simulink model "PassVeh7DOF"  (R2024b)
settings: Solver=ode14x  StartTime=0.0  StopTime=30  FixedStep=0.001  RelTol=1e-1
model workspace (MAT data in the model file):
  A_mu = 10
  B_reff = 8.386
  CONVERTER_DATA = [0 0.1 0.2 0.3 0.4 0.5 0.6 0.7 0.8 0.81 0.82 0.83 ... (63 elements, 21x3)]
  Cps = 2
  Cz = 7766.25
  DOWN_TABLE = [0 0 0 0 0 0 5 5 7.5 7.5 15 15 ... (30 elements, 6x5)]
  DOWN_TH_BP = [0 5 40 50 90 100]
  D_reff = 0.25826
  EMAP = [-40 215 245 264 264 267 267 267 267 267 -44 117 ... (110 elements, 10x11)]
  F0z = [6086.4 4324.8]
  F_reff = 0.07394
  F_zmax = 10000
  F_zmin = 100
  F_zo = 4000
  Kz = 48000
  MF : object (value not decoded)
  NCyl = 6
  NE_VEC = [800 1200 1600 2000 2400 2800 3200 3600 4000 4400 4800]
  Pstd = 101325
  R_eff = 0.298
  Rair = 287
  SUS : object (value not decoded)
  TH_VEC = [0; 20; 30; 40; 50; 60; 70; 80; 90; 100]
  TWAITdn = 1.25
  TWAITup = 0.1
  Tin = [1 2 3 4 5 6 7 8 9 10 2 2 ... (20 elements, 10x2)]
  Tstd = 293.15
  UP_TABLE = [7.5 7.5 15 25 40 40 25 25 35 45 70 80 ... (30 elements, 6x5)]
  UP_TH_BP = [0 25 35 50 90 100]
  VEH : object (value not decoded)
  V_o = 16.7
  V_xlow = 1
  Vd = 0.00346
  WH : object (value not decoded)
  a = 1.515
  alpha_max = 1.5
  alpha_min = -1.5
  b = 1.504
  c_zo = 209651
  epsilon = 0.1
  f_air = [0 0 0 0 0 0 0 0 0 0 0 0 ... (256 elements, 16x16)]
  f_co = [0 0 0 0 0 0 0 0 0 0 0 0 ... (256 elements, 16x16)]
  f_co2 = [0 0 0 0 0 0 0 0 0 0 0 0 ... (256 elements, 16x16)]
  f_eff = [352.135682859 352.135682859 320.724378192 303.655312657 295.930136708 291.240087194 291.240271258 291.240312459 291.240275452 291.240198499 291.240100781 291.240018769 ... (256 elements, 16x16)]
  f_fuel = [0 0 0 0 0 0 0 0 0 0 0 0 ... (256 elements, 16x16)]
  f_hc = [0 0 0 0 0 0 0 0 0 0 0 0 ... (256 elements, 16x16)]
  f_nox = [0 0 0 0 0 0 0 0 0 0 0 0 ... (256 elements, 16x16)]
  f_pm = [0 0 0 0 0 0 0 0 0 0 0 0 ... (256 elements, 16x16)]
  f_susp_axl_bp = [1 2]
  f_susp_dz_bp = [-4 -0.14 -0.13 -0.12 -0.11 -0.1 -0.09 -0.08 -0.07 -0.06 -0.05 -0.04 ... (31 elements, 1x31)]
  f_susp_dzdot_bp = [-4 -0.14 -0.13 -0.12 -0.11 -0.1 -0.09 -0.08 -0.07 -0.06 -0.05 -0.04 ... (31 elements, 1x31)]
  f_susp_fmz = [-213379.591456 -28099.591456 -27619.591456 -27139.591456 -26659.591456 -26179.591456 -25699.591456 -25219.591456 -24739.591456 -24259.591456 -23779.591456 -23299.591456 ... (468968 elements, 31x31x61x2x4)]
  f_susp_geom = [-0.832564012244 0.043269987756 0.045538987756 0.047807987756 0.050076987756 0.052345987756 0.054614987756 0.056883987756 0.059152987756 0.061421987756 0.063690987756 0.065959987756 ... (11346 elements, 31x61x2x3)]
  f_susp_strgdelta_bp = [-0.523598775598 -0.506145483078 -0.488692190558 -0.471238898038 -0.453785605519 -0.436332312999 -0.418879020479 -0.401425727959 -0.383972435439 -0.366519142919 -0.349065850399 -0.331612557879 ... (61 elements, 1x61)]
  f_tbrake = [0 76.8593923996 105.140482948 131.533638111 157.926793274 176.658631717 176.65727296 176.656856686 176.656879077 176.657093756 176.657404516 176.65772406 ... (256 elements, 16x16)]
  f_tbrake_n_bpt = [0 649.519052838 912.419621844 1175.32019085 1438.22075986 1701.12132886 1964.02189787 2226.92246687 2489.82303588 2752.72360489 3015.62417389 3278.5247429 ... (16 elements, 1x16)]
  f_tbrake_t_bpt = [0 34.6410161514 61.0341713143 87.4273264773 113.82048164 140.213636803 166.606791966 192.999947129 219.393102292 245.786257455 272.179412618 298.572567781 ... (16 elements, 1x16)]
  f_texh = [766.752464599 766.752464599 786.17542386 801.679939032 884.591982581 910.574397722 910.571871054 910.570774534 910.570601632 910.570821151 910.571247242 910.571639815 ... (256 elements, 16x16)]
  f_twc_eff_co = [0.17 0.25 0.45 0.99 0.99 0.99 0.99]
  f_twc_eff_hc = [0.21 0.375 0.75 0.98 0.98 0.98 0.98]
  f_twc_eff_lam = [0.909090909 0.944055944 0.979020979 1 1.013986014 1.048951049 1.083916084]
  f_twc_eff_nox = [0.98 0.98 0.98 0.97 0.05 0.02 0]
  h = 0.134
  k_z = 50
  kappa_max = 1.5
  kappa_min = -1.5
  lam_Cx = 1
  lam_Cy = 1
  lam_Cz = 1
  lam_Ex = 1
  lam_Ey = 1
  lam_F_zo = 1
  lam_Hx = 1
  lam_Hy = 1
  lam_Kxkappa = 1
  lam_Kyalpha = 1
  lam_Kygamma = 1
  lam_Kzgamma = 1
  lam_Mr = 1
  lam_Mx = 1
  lam_My = 1
  lam_S = 1
  lam_VMx = 1
  lam_Vx = 1
  lam_Vy = 1
  lam_Vykappa = 1
  lam_muV = 0
  lam_mux = 1
  lam_muy = 1
  lam_t = 1
  lam_xalpha = 1
  lam_ykappa = 1
  numWheel = 4
  p_Cx1 = 1.579
  p_Cy1 = 1.3332
  p_Dx1 = 1.0422
  p_Dx2 = -0.08285
  p_Dx3 = 0
  p_Dy1 = 0.8784
  p_Dy2 = -0.06445
  p_Dy3 = 0
  p_Ex1 = 0.11185
  p_Ex2 = 0.3127
  p_Ex3 = 0
  p_Ex4 = 0.001603
  p_Ey1 = -0.8227
  p_Ey2 = -0.6062
  p_Ey3 = 0.09825
  p_Ey4 = -6.546
  p_Ey5 = 0
  p_Fz1 = 0.7098
  p_Hx1 = 0.00021585
  p_Hx2 = 0.0011538
  p_Hy1 = -0.0018043
  p_Hy2 = 0.003518
  p_Kx1 = 21.69
  p_Kx2 = 13.774
  p_Kx3 = -0.4119
  p_Ky1 = -15.314
  p_Ky2 = 1.7044
  p_Ky3 = 0.36986
  p_Ky4 = 1.9896
  p_Ky5 = 0
  p_Ky6 = -0.9004
  p_Ky7 = -0.2328
  p_Vx1 = 1.5973e-05
  p_Vx2 = 0.0001043
  p_Vy1 = -0.006642
  p_Vy2 = 0.03597
  p_Vy3 = -0.1621
  p_Vy4 = -0.4908
  p_pmx1 = 0
  p_px1 = -0.3489
  p_px2 = 0.382
  p_px3 = -0.09634
  p_px4 = 0.06447
  p_py1 = -0.6249
  p_py2 = -0.06535
  p_py3 = -0.1668
  p_py4 = 0.2834
  p_py5 = 0
  path : object (value not decoded)
  pio = 220000
  q_Fcx = 0
  q_Fz2 = 15.4
  q_Fzy = 0
  q_reo = 0.9974
  q_sx1 = -0.007764
  q_sx10 = 0.2824
  q_sx11 = 5.349
  q_sx12 = 0
  q_sx13 = 0
  q_sx14 = 0
  q_sx2 = 1.1915
  q_sx3 = 0.013948
  q_sx4 = 4.912
  q_sx5 = 1.02
  q_sx6 = 22.83
  q_sx7 = 0.7104
  q_sx8 = -0.023393
  q_sx9 = 0.6581
  q_sy1 = 0.00702
  q_sy2 = 0
  q_sy3 = 0.001515
  q_sy4 = 8.514e-05
  q_sy5 = 0
  q_sy6 = 0
  q_sy7 = 0.9008
  q_sy8 = -0.4089
  q_v1 = 0.0007742
  q_v2 = 0.04667
  r_Bx1 = 12.531
  r_Bx2 = 9.532
  r_Bx3 = 0
  r_By1 = 10.615
  r_By2 = 7.705
  r_By3 = 3.433e-06
  r_By4 = 0
  r_Cx1 = 1.019
  r_Cy1 = 1.0585
  r_Ex1 = -0.4487
  r_Ex2 = -0.4726
  r_Ey1 = 0.3132
  r_Ey2 = 7.63e-06
  r_Hx1 = 0.0002374
  r_Hy1 = 0.011646
  r_Hy2 = 7.63e-06
  r_Vy1 = 0.05654
  r_Vy2 = 7.63e-06
  r_Vy3 = 0
  r_Vy4 = 99.9
  r_Vy5 = 2
  r_Vy6 = 15.814
  r_o = 0.3135
  reqTmaxT = [nan 0.285774810084 0.647179872268 nan nan nan nan nan nan nan nan nan ... (168 elements, 21x8)]
  vehSpd = [0 2.77777777778 5.55555555556 8.33333333333 11.1111111111 13.8888888889 16.6666666667 19.4444444444 22.2222222222 25 27.7777777778 30.5555555556 ... (21 elements, 1x21)]
  vehWidth = 2
  w = 1
symbols that are objects in the model workspace (value not decoded): VEH
undefined symbols (not defined in the file or in its folder): Fzz, Fzzdot, InertFrm, pFz, psi, vdyntiremask, x_o, zdotFz, zFz
libraries: simulink x4, sharedTrackingLibrary x1, mcbcontrolslib x1
(part 8 of 24)

== system PassVeh7DOF/Longitudinal Wheels 4DOF/Tires/Fiala/Fiala Tire/Vertical DOF ==
  "GroundInput " : Inport
  "Fext " : Inport  Port=2
  rho : Inport  Port=3
  "GndFz " : Inport  Port=4
  Prs : Inport  Port=5
  External : Subsystem  VariantControl=vertType==3
  Mapped Vertical DOF : Subsystem  VariantControl=vertType==2
  None : Subsystem  VariantControl=vertType==1
  Vertical Wheel and Unsprung Mass Response : Subsystem  VariantControl=vertType==4  mask{m=MASS, bz=VERTICAL_DAMPING, zo=zo, zdoto=zdoto, g=GRAVITY, ReMax=UNLOADED_RADIUS}
      mask prompts: m "Unsprung mass [kg]"; bz "Vertical damping [N*m/s]"; zo "Initial deflection [m]"; zdoto "Initial velocity [m/s]"; g "Gravitational acceleration [m/s^2]"; ReMax "Maximum unloaded radius [m]:"
  RadialDeflct : Outport  VectorParamsAs1DForOutWhenUnconnected=off
  " z" : Outport  Port=2  VectorParamsAs1DForOutWhenUnconnected=off
  " zdot" : Outport  Port=3  VectorParamsAs1DForOutWhenUnconnected=off
  GndFz : Outport  Port=4  VectorParamsAs1DForOutWhenUnconnected=off

== system PassVeh7DOF/Longitudinal Wheels 4DOF/Tires/Fiala/Fiala Tire/Wheel Module ==
  BrkPrs : Inport
  AxlTrq : Inport  Port=2
  TireFdbk : Inport  Port=3
  RadialDeflct : Inport  Port=4
  Add1 : Sum  Inputs=--+
  Add2 : Sum  Inputs=-+
  Brakes : Subsystem  Variant=on  VariantControlMode=label  LabelModeActiveChoice=Disk  mask{aMode=aMode}
  Bus Selector1 : BusSelector  OutputSignals=My,Fx
  Clutch : Subsystem  Variant=on  VariantControlMode=label  VariantControl=Choice  LabelModeActiveChoice=0
  Constant9 : Constant  Value=UNLOADED_RADIUS
  Friction Model : Subsystem
  Product3 : Product  Inputs=**
  Reshape : Reshape
  Saturation : Saturate  UpperLimit=inf  LowerLimit=0  ZeroCross=off
  Terminator1 : Terminator
  Terminator3 : Terminator
  MyBrk : Outport  VectorParamsAs1DForOutWhenUnconnected=off
  Omega : Outport  Port=2  VectorParamsAs1DForOutWhenUnconnected=off
  wires:
  Reshape/1 -> Clutch/1(Tout)
  Product3/1 -> Add1/3
  AxlTrq/1 -> Add1/1
  RadialDeflct/1 -> Add2/1
  Friction Model/2(Tfmaxk) -> Clutch/3(Tfmaxk)
  Friction Model/1(Tfmaxs) -> Clutch/2(Tfmaxs)
  Add1/1 -> Reshape/1
  Clutch/3(Myb) -> Terminator1/1
  Clutch/2(Omegadot) -> Terminator3/1
  Clutch/1(Omega) -> Brakes/2(Omega), Omega/1
  Saturation/1 -> Product3/2
  Brakes/1(MyBrk) -> Friction Model/1(Brake torque), MyBrk/1
  Add2/1 -> Saturation/1
  Constant9/1 -> Add2/2
  BrkPrs/1 -> Brakes/1(BrkPrs)
  Bus Selector1/2 -> Product3/1  "<Fx>"
  Bus Selector1/1 -> Add1/2  "<My>"
  TireFdbk/1 -> Bus Selector1/1

== system PassVeh7DOF/Longitudinal Wheels 4DOF/Tires/MF/Combined Slip Wheel 2DOF/Bus Routing ==
  BrkPrs : Inport
  BrkTrq : Inport  Port=2
  omega : Inport  Port=3
  FLong : Inport  Port=4
  Flat : Inport  Port=5
  FzTire : Inport  Port=6
  MOver : Inport  Port=7
  MRoll : Inport  Port=8
  MAlign : Inport  Port=9
  Re : Inport  Port=10
  Kappa : Inport  Port=11
  Alpha : Inport  Port=12
  a : Inport  Port=13
  b : Inport  Port=14
  RL : Inport  Port=15
  RadialDeflct : Inport  Port=16
  WhlTrq : Inport  Port=17
  z : Inport  Port=18
  zdot : Inport  Port=19
  AxlTrq : Inport  Port=20
  Vx : Inport  Port=21
  Vy : Inport  Port=22
  Gamma : Inport  Port=23
  psidot : Inport  Port=24
  Prs : Inport  Port=25
  Gnd : Inport  Port=26
  FNormal : Inport  Port=27
  Bus Creator : BusCreator  Inputs=27
  Signal Copy : SignalConversion  OverrideOpt=off
  Signal Specification{,3,6..7,22..23} (6 alike) : SignalSpecification  Unit=m
  Signal Specification1 : SignalSpecification  Unit=1
  Signal Specification{5,8,15..17} (5 alike) : SignalSpecification  Unit=N*m
  Signal Specification18 : SignalSpecification  Unit=N
  Signal Specification19 : SignalSpecification  Unit=N
  Signal Specification2 : SignalSpecification  Unit=rad
  Signal Specification20 : SignalSpecification  Unit=N
  Signal Specification21 : SignalSpecification  Unit=rad/s
  Signal Specification4 : SignalSpecification  Unit=m/s
  Info : Outport  VectorParamsAs1DForOutWhenUnconnected=off
  Omega : Outport  Port=2  Unit=rad/s  VectorParamsAs1DForOutWhenUnconnected=off
  Fx : Outport  Port=3  Unit=N  VectorParamsAs1DForOutWhenUnconnected=off
  Fy : Outport  Port=4  Unit=N  VectorParamsAs1DForOutWhenUnconnected=off
  Fz : Outport  Port=5  Unit=N  VectorParamsAs1DForOutWhenUnconnected=off
  Mx : Outport  Port=6  Unit=N*m  VectorParamsAs1DForOutWhenUnconnected=off
  My : Outport  Port=7  Unit=N*m  VectorParamsAs1DForOutWhenUnconnected=off
  Mz : Outport  Port=8  Unit=N*m  VectorParamsAs1DForOutWhenUnconnected=off
  wires:
  Signal Specification5/1 -> Bus Creator/21  "BrkTrq"
  psidot/1 -> Bus Creator/20  "psidot"
  Gamma/1 -> Bus Creator/19  "Gamma"
  Signal Specification8/1 -> Bus Creator/18  "WhlTrq"
  Signal Specification7/1 -> Bus Creator/17  "RadialDeflct"
  Signal Specification6/1 -> Bus Creator/16  "RL"
  RL/1 -> Signal Specification6/1
  RadialDeflct/1 -> Signal Specification7/1
  WhlTrq/1 -> Signal Specification8/1
  MRoll/1 -> Signal Specification16/1
  FzTire/1 -> Signal Copy/1
  Signal Copy/1 -> Signal Specification18/1
  Prs/1 -> Bus Creator/27  "Prs"
  Gnd/1 -> Bus Creator/25  "Gnd"
  Signal Specification18/1 -> Bus Creator/26  "GndFz"
  BrkPrs/1 -> Bus Creator/22  "BrkPrs"
  Vy/1 -> Bus Creator/10  "Vy"
  Vx/1 -> Bus Creator/9  "Vx"
  AxlTrq/1 -> Bus Creator/1  "AxlTrq"
  BrkTrq/1 -> Signal Specification5/1
  Kappa/1 -> Signal Specification1/1
  z/1 -> Signal Specification3/1
  zdot/1 -> Signal Specification4/1
  Re/1 -> Signal Specification/1
  b/1 -> Signal Specification22/1
  Flat/1 -> Signal Specification19/1
  MAlign/1 -> Signal Specification15/1
  Signal Specification22/1 -> Bus Creator/15  "b"
  Signal Specification23/1 -> Bus Creator/14  "a"
  Signal Specification20/1 -> Fx/1, Bus Creator/3  "Fx"
  Signal Specification2/1 -> Bus Creator/13  "Alpha"
  omega/1 -> Signal Specification21/1
  Signal Specification16/1 -> Bus Creator/7, My/1  "My"
  Signal Specification19/1 -> Bus Creator/4, Fy/1  "Fy"
  FLong/1 -> Signal Specification20/1
  Signal Specification1/1 -> Bus Creator/12  "Kappa"
  MOver/1 -> Signal Specification17/1
  Signal Specification17/1 -> Bus Creator/6, Mx/1  "Mx"
  Bus Creator/1 -> Info/1
  Signal Specification/1 -> Bus Creator/11  "Re"
  Signal Specification15/1 -> Bus Creator/8, Mz/1  "Mz"
  FNormal/1 -> Bus Creator/5, Fz/1  "Fz"
  Signal Specification21/1 -> Omega/1, Bus Creator/2  "Omega"
  Signal Specification4/1 -> Bus Creator/24  "zdot"
  Alpha/1 -> Signal Specification2/1
  a/1 -> Signal Specification23/1
  Signal Specification3/1 -> Bus Creator/23  "z"

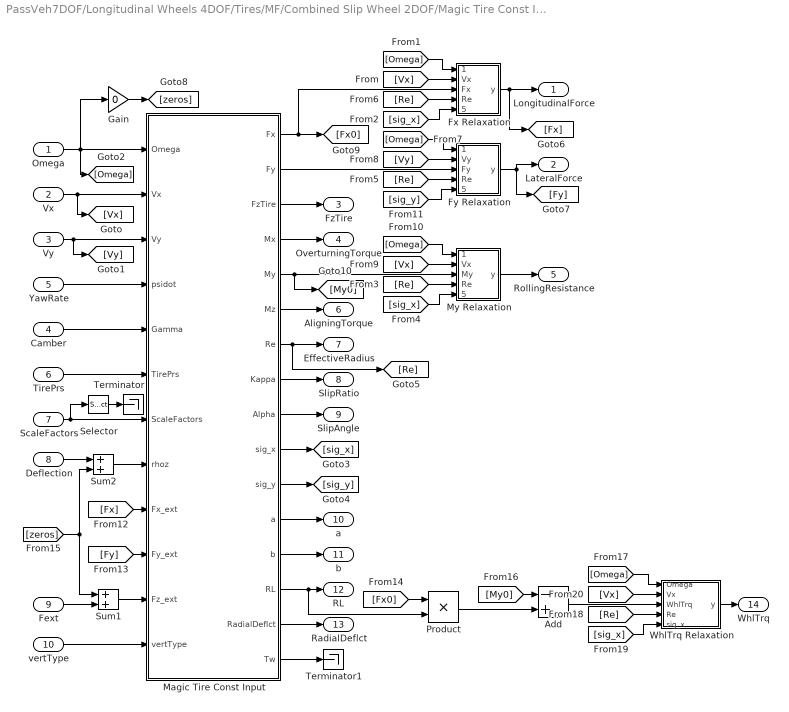
== system PassVeh7DOF/Longitudinal Wheels 4DOF/Tires/MF/Combined Slip Wheel 2DOF/Magic Tire Const Input ==
  Omega : Inport
  Vx : Inport  Port=2
  Vy : Inport  Port=3
  Camber : Inport  Port=4
  YawRate : Inport  Port=5
  TirePrs : Inport  Port=6
  ScaleFactors : Inport  Port=7
  Deflection : Inport  Port=8
  Fext : Inport  Port=9
  vertType : Inport  Port=10
  Add : Sum  Inputs=-+
  Fx Relaxation : Subsystem
  Fy Relaxation : Subsystem
  Gain : Gain  Gain=0
  Magic Tire Const Input : MATLAB Function
  My Relaxation : Subsystem
  Product : Product
  Selector : Selector  NumberOfDimensions=2  InputPortWidth=3  IndexOptions=Index vector (dialog),Select all  Indices=[1:27],1  OutputSizes=1,1
  Sum1 : Sum
  Sum2 : Sum
  Terminator : Terminator
  Terminator1 : Terminator
  WhlTrq Relaxation : Subsystem
  LongitudinalForce : Outport  VectorParamsAs1DForOutWhenUnconnected=off
  LateralForce : Outport  Port=2  VectorParamsAs1DForOutWhenUnconnected=off
  FzTire : Outport  Port=3  VectorParamsAs1DForOutWhenUnconnected=off
  OverturningTorque : Outport  Port=4  VectorParamsAs1DForOutWhenUnconnected=off
  RollingResistance : Outport  Port=5  VectorParamsAs1DForOutWhenUnconnected=off
  AligningTorque : Outport  Port=6  VectorParamsAs1DForOutWhenUnconnected=off
  EffectiveRadius : Outport  Port=7  VectorParamsAs1DForOutWhenUnconnected=off
  SlipRatio : Outport  Port=8  VectorParamsAs1DForOutWhenUnconnected=off
  SlipAngle : Outport  Port=9  VectorParamsAs1DForOutWhenUnconnected=off
  a : Outport  Port=10  VectorParamsAs1DForOutWhenUnconnected=off
  b : Outport  Port=11  VectorParamsAs1DForOutWhenUnconnected=off
  RL : Outport  Port=12
  RadialDeflct : Outport  Port=13
  WhlTrq : Outport  Port=14
  wires:
  Add/1 -> WhlTrq Relaxation/3(WhlTrq)
  WhlTrq Relaxation/1(y) -> WhlTrq/1
  [Re] -> WhlTrq Relaxation/4(Re)
  [Vx] -> WhlTrq Relaxation/2(Vx)
  [sig_x] -> WhlTrq Relaxation/5(sig_x)
  [Omega] -> WhlTrq Relaxation/1(Omega)
  [My0] -> Add/1
  Deflection/1 -> Sum2/1
  Sum2/1 -> Magic Tire Const Input/8(rhoz)
  [zeros] -> Sum2/2, Sum1/1
  Sum1/1 -> Magic Tire Const Input/11(Fz_ext)
  Fext/1 -> Sum1/2
  Gain/1 -> [zeros]
  Product/1 -> Add/2
  [Fx0] -> Product/1
  Magic Tire Const Input/16(Tw) -> Terminator1/1
  Magic Tire Const Input/15(RadialDeflct) -> RadialDeflct/1
  Magic Tire Const Input/14(RL) -> RL/1, Product/2
  Selector/1 -> Terminator/1
  vertType/1 -> Magic Tire Const Input/12(vertType)
  [Fy] -> Magic Tire Const Input/10(Fy_ext)
  [Fx] -> Magic Tire Const Input/9(Fx_ext)
  Magic Tire Const Input/1(Fx) -> [Fx0], Fx Relaxation/3(Fx)
  [sig_y] -> Fy Relaxation/5(sig_y)
  [Omega] -> My Relaxation/1(Omega)
  [Vx] -> My Relaxation/2(Vx)
  [Vy] -> Fy Relaxation/2(Vy)
  [Omega] -> Fy Relaxation/1(Omega)
  [Re] -> Fx Relaxation/4(Re)
  [Re] -> Fy Relaxation/4(Re)
  [sig_x] -> My Relaxation/5(sig_x)
  [Re] -> My Relaxation/4(Re)
  [sig_x] -> Fx Relaxation/5(sig_x)
  Magic Tire Const Input/11(sig_y) -> [sig_y]
  Magic Tire Const Input/10(sig_x) -> [sig_x]
  [Omega] -> Fx Relaxation/1(Omega)
  [Vx] -> Fx Relaxation/2(Vx)
  Fy Relaxation/1(y) -> [Fy], LateralForce/1
  Magic Tire Const Input/12(a) -> a/1
  Magic Tire Const Input/13(b) -> b/1
  Magic Tire Const Input/5(My) -> My Relaxation/3(My), [My0]
  Vy/1 -> Magic Tire Const Input/3(Vy), [Vy]
  Vx/1 -> [Vx], Magic Tire Const Input/2(Vx)
  My Relaxation/1(y) -> RollingResistance/1
  Fx Relaxation/1(y) -> [Fx], LongitudinalForce/1
  Magic Tire Const Input/7(Re) -> [Re], EffectiveRadius/1
  Magic Tire Const Input/2(Fy) -> Fy Relaxation/3(Fy)
  Magic Tire Const Input/9(Alpha) -> SlipAngle/1
  Magic Tire Const Input/8(Kappa) -> SlipRatio/1
  Magic Tire Const Input/6(Mz) -> AligningTorque/1
  Magic Tire Const Input/4(Mx) -> OverturningTorque/1
  ScaleFactors/1 -> Selector/1, Magic Tire Const Input/7(ScaleFactors)
  TirePrs/1 -> Magic Tire Const Input/6(TirePrs)
  Camber/1 -> Magic Tire Const Input/5(Gamma)
  YawRate/1 -> Magic Tire Const Input/4(psidot)
  Omega/1 -> [Omega], Magic Tire Const Input/1(Omega), Gain/1
  Magic Tire Const Input/3(FzTire) -> FzTire/1

== system PassVeh7DOF/Longitudinal Wheels 4DOF/Tires/MF/Combined Slip Wheel 2DOF/Vertical DOF ==
  "GroundInput " : Inport
  "Fext " : Inport  Port=2
  rho : Inport  Port=3
  Prs : Inport  Port=4
  Omega : Inport  Port=5
  Gamma : Inport  Port=6
  Fx_ext : Inport  Port=7
  Fy_ext : Inport  Port=8
  "GndFz " : Inport  Port=9
  ScaleFctrs : Inport  Port=10
  External : Subsystem  VariantControl=vertType==3
  Mapped Vertical DOF : Subsystem  VariantControl=vertType==4
  None : Subsystem  VariantControl=vertType==1
  Vertical Wheel and Unsprung Mass Response : Subsystem  VariantControl=vertType==2  mask{m=MASS, bz=VERTICAL_DAMPING, zo=zo, zdoto=zdoto, g=GRAVITY, ReMax=UNLOADED_RADIUS}
      mask prompts: m "Unsprung mass [kg]"; bz "Vertical damping [N*m/s]"; zo "Initial deflection [m]"; zdoto "Initial velocity [m/s]"; g "Gravitational acceleration [m/s^2]"; ReMax "Maximum unloaded radius [m]:"
  " RadialDeflct" : Outport  VectorParamsAs1DForOutWhenUnconnected=off
  GndFz : Outport  Port=2  VectorParamsAs1DForOutWhenUnconnected=off
  " z" : Outport  Port=3  VectorParamsAs1DForOutWhenUnconnected=off
  " zdot" : Outport  Port=4  VectorParamsAs1DForOutWhenUnconnected=off

== system PassVeh7DOF/Longitudinal Wheels 4DOF/Tires/MF/Combined Slip Wheel 2DOF/Wheel Module ==
  BrkPrs : Inport
  AxlTrq : Inport  Port=2
  TireFdbk : Inport  Port=3
  RadialDeflct : Inport  Port=4
  Add1 : Sum  Inputs=--+
  Add2 : Sum  Inputs=-+
  Brakes : Subsystem  Variant=on  VariantControlMode=label  LabelModeActiveChoice=Disk  mask{aMode=aMode}
  Bus Selector1 : BusSelector  OutputSignals=My,Fx
  Clutch : Subsystem  Variant=on  VariantControlMode=label  VariantControl=Choice  LabelModeActiveChoice=0
  Constant9 : Constant  Value=UNLOADED_RADIUS
  Friction Model : Subsystem
  Product3 : Product  Inputs=**
  Reshape : Reshape
  Saturation : Saturate  UpperLimit=inf  LowerLimit=0  ZeroCross=off
  Terminator1 : Terminator
  Terminator3 : Terminator
  MyBrk : Outport  VectorParamsAs1DForOutWhenUnconnected=off
  Omega : Outport  Port=2  VectorParamsAs1DForOutWhenUnconnected=off
  wires:
  Reshape/1 -> Clutch/1(Tout)
  Product3/1 -> Add1/3
  AxlTrq/1 -> Add1/1
  RadialDeflct/1 -> Add2/1
  Friction Model/2(Tfmaxk) -> Clutch/3(Tfmaxk)
  Friction Model/1(Tfmaxs) -> Clutch/2(Tfmaxs)
  Add1/1 -> Reshape/1
  Clutch/3(Myb) -> Terminator1/1
  Clutch/2(Omegadot) -> Terminator3/1
  Clutch/1(Omega) -> Brakes/2(Omega), Omega/1
  Saturation/1 -> Product3/2
  Brakes/1(MyBrk) -> Friction Model/1(Brake torque), MyBrk/1
  Add2/1 -> Saturation/1
  Constant9/1 -> Add2/2
  BrkPrs/1 -> Brakes/1(BrkPrs)
  Bus Selector1/2 -> Product3/1  "<Fx>"
  Bus Selector1/1 -> Add1/2  "<My>"
  TireFdbk/1 -> Bus Selector1/1

== system PassVeh7DOF/Longitudinal Wheels 4DOF/Tires/MF/Combined Slip Wheel 2DOF/a_cmd ==
  note: $\alpha_{\text{cmd}} = \arctan\left( \frac{v_y + ar}{v_x} \right) - \delta$
  Vx : Inport
  Vy : Inport  Port=2
  WhlAng : Inport  Port=3
  YawRate : Inport  Port=4
  Add1 : Sum
  Gain : Gain  Gain=VEH.FrontAxlePositionfromCG
  Subtract : Sum  Inputs=+-
  atan2 : mcbcontrolslib/atan2  ApproximationMethod=None  NumberOfIterations=11  NumberOfDataPoints=16  InterpMethod=Flat  outputUnit=Radians  TableDataTypeStr=Inherit: Inherit via input
      settings: LibrarySourceBlock=mcblib/Controls/Math Transforms/atan2
  alphacmd : Outport
  wires:
  Subtract/1 -> alphacmd/1
  WhlAng/1 -> Subtract/2
  Add1/1 -> atan2/1
  Vy/1 -> Add1/1
  atan2/1 -> Subtract/1
  Gain/1 -> Add1/2
  YawRate/1 -> Gain/1
  Vx/1 -> atan2/2

== system PassVeh7DOF/Longitudinal Wheels 4DOF/Tires/MF/Combined Slip Wheel 2DOF/k_cmd ==
  note: $\kappa_{\text{cmd}} = \frac{R_{\text{eff}} \cdot \omega - v_x}{\max(|v_x|, 0.1)}$$
  Omega : Inport
  Vx : Inport  Port=2
  Abs : Abs  SaturateOnIntegerOverflow=off
  Constant : Constant  Value=0.1
  Divide : Product  Inputs=*/
  Gain : Gain  Gain=R_eff
  Max : MinMax  Function=max  Inputs=2
  Subtract : Sum  Inputs=+-
  k_cmd : Outport
  wires:
  Gain/1 -> Subtract/1
  Omega/1 -> Gain/1
  Max/1 -> Divide/2
  Constant/1 -> Max/2
  Vx/1 -> Subtract/2, Abs/1
  Subtract/1 -> Divide/1
  Abs/1 -> Max/1
  Divide/1 -> k_cmd/1

== system PassVeh7DOF/Longitudinal Wheels 4DOF/Veh2Tire/Wheel to Body Transform/Rotation Angles to Direction Cosine Matrix/Create 3x3 Matrix ==
  M11 : Inport  PortDimensions=1
  M12 : Inport  Port=2  PortDimensions=1
  M13 : Inport  Port=3  PortDimensions=1
  M21 : Inport  Port=4  PortDimensions=1
  M22 : Inport  Port=5  PortDimensions=1
  M23 : Inport  Port=6  PortDimensions=1
  M31 : Inport  Port=7  PortDimensions=1
  M32 : Inport  Port=8  PortDimensions=1
  M33 : Inport  Port=9  PortDimensions=1
  Reshape (9) to [3x3] column-major : Reshape  OutputDimensionality=Customize  OutputDimensions=[3,3]
  Vector Concatenate : Concatenate  NumInputs=9
  Matrix : Outport  PortDimensions=[3 3]  VectorParamsAs1DForOutWhenUnconnected=off
  wires:
  M33/1 -> Vector Concatenate/9
  M23/1 -> Vector Concatenate/8
  M13/1 -> Vector Concatenate/7
  M32/1 -> Vector Concatenate/6
  Reshape (9) to [3x3] column-major/1 -> Matrix/1
  M22/1 -> Vector Concatenate/5
  M12/1 -> Vector Concatenate/4
  M31/1 -> Vector Concatenate/3
  M21/1 -> Vector Concatenate/2
  M11/1 -> Vector Concatenate/1
  Vector Concatenate/1 -> Reshape (9) to [3x3] column-major/1

== system PassVeh7DOF/Longitudinal Wheels 4DOF/Velocity and Vertical Load/Bicycle/Bicycle Fz/Cont LPF ==
  u : Inport
  Constant : Constant  Value=wc
  Divide : Product  Inputs=**
  FixPt Data Type Duplicate1 : DataTypeDuplicate  DisableCoverage=on  NumInputPorts=4
  Integrator1 : Integrator
  Sum : Sum  Inputs=|+-
  y : Outport  VectorParamsAs1DForOutWhenUnconnected=off
  wires:
  Constant/1 -> Divide/2
  [y] -> FixPt Data Type Duplicate1/3
  [wumy] -> FixPt Data Type Duplicate1/4
  [umy] -> FixPt Data Type Duplicate1/2
  [u] -> FixPt Data Type Duplicate1/1
  Integrator1/1 -> y/1, [y], Sum/2
  u/1 -> [u], Sum/1
  Sum/1 -> [umy], Divide/1
  Divide/1 -> [wumy], Integrator1/1

== system PassVeh7DOF/Longitudinal Wheels 4DOF/Velocity and Vertical Load/Dual/Dual Fz/Cont LPF ==
  u : Inport
  Constant : Constant  Value=wc
  Divide : Product  Inputs=**
  FixPt Data Type Duplicate1 : DataTypeDuplicate  DisableCoverage=on  NumInputPorts=4
  Integrator1 : Integrator
  Sum : Sum  Inputs=|+-
  y : Outport  VectorParamsAs1DForOutWhenUnconnected=off
  wires:
  Constant/1 -> Divide/2
  [y] -> FixPt Data Type Duplicate1/3
  [wumy] -> FixPt Data Type Duplicate1/4
  [umy] -> FixPt Data Type Duplicate1/2
  [u] -> FixPt Data Type Duplicate1/1
  Integrator1/1 -> y/1, [y], Sum/2
  u/1 -> [u], Sum/1
  Sum/1 -> [umy], Divide/1
  Divide/1 -> [wumy], Integrator1/1

== system PassVeh7DOF/Vehicle Body 3DOF External Longitudinal Wheels/Bicycle/Vehicle Body 3DOF Single Track/Cy/Cy const ==
  Cyf : Constant  Value=Cy_f
  Cyr : Constant  Value=Cy_r
  Cy_f : Outport  VectorParamsAs1DForOutWhenUnconnected=off
  Cy_r : Outport  Port=2  VectorParamsAs1DForOutWhenUnconnected=off
  wires:
  Cyr/1 -> Cy_r/1
  Cyf/1 -> Cy_f/1

== system PassVeh7DOF/Vehicle Body 3DOF External Longitudinal Wheels/Bicycle/Vehicle Body 3DOF Single Track/Cy/Cy const dual ==
  Cyf : Constant  Value=Cy_f
  Cyr : Constant  Value=Cy_r
  Vector Concatenate1 : Concatenate
  Vector Concatenate2 : Concatenate  ConcatenateDimension=2
  Cy_f : Outport  VectorParamsAs1DForOutWhenUnconnected=off
  Cy_r : Outport  Port=2  VectorParamsAs1DForOutWhenUnconnected=off
  wires:
  Cyf/1 -> Vector Concatenate2/2, Vector Concatenate2/1
  Cyr/1 -> Vector Concatenate1/2, Vector Concatenate1/1
  Vector Concatenate2/1 -> Cy_f/1
  Vector Concatenate1/1 -> Cy_r/1

== system PassVeh7DOF/Vehicle Body 3DOF External Longitudinal Wheels/Bicycle/Vehicle Body 3DOF Single Track/Cy/Cy table ==
  alpha_f : Inport
  alpha_r : Inport  Port=2
  Cy_f(alpha_f) : Lookup_n-D  NumberOfTableDimensions=1  BreakpointsForDimension1=alpha_f_brk  Table=Cy_f_data  ExtrapMethod=Clip  InternalRulePriority=Speed  RndMeth=Simplest
  Cy_r(alpha_r) : Lookup_n-D  NumberOfTableDimensions=1  BreakpointsForDimension1=alpha_r_brk  Table=Cy_r_data  ExtrapMethod=Clip  InternalRulePriority=Speed  RndMeth=Simplest
  Cy_f : Outport  VectorParamsAs1DForOutWhenUnconnected=off
  Cy_r : Outport  Port=2  VectorParamsAs1DForOutWhenUnconnected=off
  wires:
  alpha_r/1 -> Cy_r(alpha_r)/1
  alpha_f/1 -> Cy_f(alpha_f)/1
  Cy_r(alpha_r)/1 -> Cy_r/1
  Cy_f(alpha_f)/1 -> Cy_f/1

== system PassVeh7DOF/Vehicle Body 3DOF External Longitudinal Wheels/Bicycle/Vehicle Body 3DOF Single Track/Cy/Cy table dual ==
  alpha_f : Inport
  alpha_r : Inport  Port=2
  For Each Subsystem : Subsystem  TreatAsAtomicUnit=on
  Cy_f : Outport  VectorParamsAs1DForOutWhenUnconnected=off
  Cy_r : Outport  Port=2  VectorParamsAs1DForOutWhenUnconnected=off
  wires:
  alpha_r/1 -> For Each Subsystem/2(alpha_r)
  alpha_f/1 -> For Each Subsystem/1(alpha_f)
  For Each Subsystem/2(Cy_r) -> Cy_r/1
  For Each Subsystem/1(Cy_f) -> Cy_f/1

== system PassVeh7DOF/Vehicle Body 3DOF External Longitudinal Wheels/Bicycle/Vehicle Body 3DOF Single Track/Drag/Drag Force ==
  Body Axis Vel : Inport
  Body Axis Wind : Inport  Port=2
  T : Inport  Port=3  OutMin=1
  .5.*A.*Pabs./R./T : Gain  Gain=.5.*A.*Pabs./R
  4 : Gain  Gain=[4.*ones(2,1); 0]
  Add1 : Sum  Inputs=+-
  Add2 : Sum  Inputs=+-
  Constant : Constant  Value=Cd
  Constant1 : Constant  Value=Cl
  Constant2 : Constant  Value=Cpm
  Constant3 : Constant  Value=Lcpm
  Constant4 : Constant  Value=[0; 0; 1]
  Crm : Lookup_n-D  NumberOfTableDimensions=1  BreakpointsForDimension1=[-1 1]  Table=[0 0]  InternalRulePriority=Speed  RndMeth=Simplest
  Cs : Lookup_n-D  NumberOfTableDimensions=1  BreakpointsForDimension1=beta_w  Table=Cs  ExtrapMethod=Clip  InternalRulePriority=Speed  RndMeth=Simplest
  Cym : Lookup_n-D  NumberOfTableDimensions=1  BreakpointsForDimension1=beta_w  Table=Cym  InternalRulePriority=Speed  RndMeth=Simplest
  Demux : Demux  Outputs=2
  Product{,2..5} (5 alike) : Product
  Product1 : Product  Inputs=**/
  Selector : Selector  InputPortWidth=3  IndexOptions=Index vector (dialog)  Indices=[2 1]  OutputSizes=1
  Selector1 : Selector  InputPortWidth=3  IndexOptions=Index vector (dialog)  Indices=[1]  OutputSizes=1
  Selector2 : Selector  InputPortWidth=6  IndexOptions=Index vector (dialog)  Indices=[4:6]  OutputSizes=1
  Selector3 : Selector  InputPortWidth=6  IndexOptions=Index vector (dialog)  Indices=[1:3]  OutputSizes=1
  Sqrt : Sqrt
  Sum of Elements : Sum  Inputs=+
  Tanh : Trigonometry  Operator=tanh
  Trigonometric Function : Trigonometry  Operator=atan2  OutputSignalType=real
  Vector Concatenate : Concatenate  NumInputs=6
  Fd : Outport  VectorParamsAs1DForOutWhenUnconnected=off
  Md : Outport  Port=2  VectorParamsAs1DForOutWhenUnconnected=off
  wires:
  Body Axis Wind/1 -> Add1/2
  Body Axis Vel/1 -> Add1/1
  [windDir] -> Selector1/1
  Demux/2 -> Trigonometric Function/2
  Product/1 -> Sum of Elements/1
  Constant/1 -> Vector Concatenate/1
  Trigonometric Function/1 -> Crm/1, Cym/1, Cs/1
  T/1 -> Product1/3
  Selector1/1 -> Product5/1
  Crm/1 -> Vector Concatenate/4
  Selector3/1 -> Product3/2
  Selector2/1 -> Product4/1
  Constant2/1 -> Product5/2
  Sqrt/1 -> Product2/1, Product2/2
  Product4/1 -> Md/1
  Product2/1 -> Product1/1
  Demux/1 -> Trigonometric Function/1
  Product3/1 -> Fd/1
  Cs/1 -> Vector Concatenate/2
  Vector Concatenate/1 -> Product1/2
  Selector/1 -> Demux/1
  Sum of Elements/1 -> Sqrt/1
  4/1 -> Tanh/1
  Cym/1 -> Vector Concatenate/6
  .5.*A.*Pabs./R./T/1 -> Selector3/1, Selector2/1
  Tanh/1 -> [windDir], Add2/1
  Product5/1 -> Vector Concatenate/5
  Constant4/1 -> Add2/2
  Constant1/1 -> Vector Concatenate/3
  Add2/1 -> Product3/1
  Add1/1 -> Selector/1, Product/2, Product/1, 4/1
  Constant3/1 -> Product4/2
  Product1/1 -> .5.*A.*Pabs./R./T/1

== system PassVeh7DOF/Vehicle Body 3DOF External Longitudinal Wheels/Bicycle/Vehicle Body 3DOF Single Track/Drag/inertial2body ==
  psi : Inport
  WindXYZ : Inport  Port=2
  Add : Sum
  Add1 : Sum  Inputs=-+
  Demux1 : Demux  Outputs=3
  Product{,1..3} (4 alike) : Product
  Trigonometric Function : Trigonometry  Operator=sincos
  Vector Concatenate2 : Concatenate  NumInputs=3
  Windxyz : Outport  VectorParamsAs1DForOutWhenUnconnected=off
  wires:
  psi/1 -> Trigonometric Function/1
  WindXYZ/1 -> Demux1/1
  Product1/1 -> Add/2
  Demux1/3 -> Vector Concatenate2/3
  Product3/1 -> Add/1
  Add/1 -> Vector Concatenate2/1
  Add1/1 -> Vector Concatenate2/2
  Vector Concatenate2/1 -> Windxyz/1
  Product/1 -> Add1/1
  Product2/1 -> Add1/2
  Trigonometric Function/1 -> Product/1, Product1/1
  Trigonometric Function/2 -> Product2/1, Product3/1
  Demux1/1 -> Product/2, Product3/2
  Demux1/2 -> Product1/2, Product2/2

== system PassVeh7DOF/Vehicle Body 3DOF External Longitudinal Wheels/Bicycle/Vehicle Body 3DOF Single Track/Signal Routing/Signal Routing ==
  y : Inport  PortDimensions=3
  Fbody : Inport  Port=2
  MTotal : Inport  Port=3
  FOut : Inport  Port=4  PortDimensions=6
  FTire : Inport  Port=5
  Fg : Inport  Port=6
  FDrag : Inport  Port=7
  MDrag : Inport  Port=8
  FExt : Inport  Port=9
  MExt : Inport  Port=10
  x : Inport  Port=11
  WhlAngF : Inport  Port=12
  WhlAngR : Inport  Port=13
  Fh : Inport  Port=14
  Mh : Inport  Port=15
  Xo : Inport  Port=16
  Bus Creator17 : BusCreator  Inputs=3
  Bus Selector : BusSelector  OutputSignals=Ang.psi
  Bus Selector1 : BusSelector  OutputSignals=InertFrm
  Bus Selector2 : BusSelector  OutputSignals=BdyFrm
  Demux : Demux  Outputs=3
  Forces 3DOF : Subsystem  VariantControl=2
  Ground : Ground
  Lateral 3DOF : Subsystem  VariantControl=3  mask(Longitudinal 3DOF){aMode=aMode}
  Moments : Subsystem
  Power : Subsystem  VariantControl=3
  Selector : Selector  IndexOptions=Index vector (dialog)  Indices=[1,2,4]  OutputSizes=1
  Signal Specification1 : SignalSpecification  Unit=m/s
  Signal Specification15 : SignalSpecification  Unit=m/s
  Signal Specification2 : SignalSpecification  Unit=rad/s
  Vector Concatenate : Concatenate
  Vector Concatenate1 : Concatenate
  state2bus : Subsystem
  Info : Outport  VectorParamsAs1DForOutWhenUnconnected=off
  xdot : Outport  Port=2  VectorParamsAs1DForOutWhenUnconnected=off
  ydot : Outport  Port=3  VectorParamsAs1DForOutWhenUnconnected=off
  psi : Outport  Port=4  VectorParamsAs1DForOutWhenUnconnected=off
  r : Outport  Port=5  VectorParamsAs1DForOutWhenUnconnected=off
  FzF : Outport  Port=6  VectorParamsAs1DForOutWhenUnconnected=off
  FzR : Outport  Port=7  VectorParamsAs1DForOutWhenUnconnected=off
  wires:
  Fh/1 -> Forces 3DOF/7(Fh)
  FDrag/1 -> Forces 3DOF/2(Fdrag)
  Mh/1 -> Moments/4(Mh)  "Mh"
  Bus Selector/1 -> psi/1  "<psi>"
  Ground/1 -> Power/5(Fsusp)
  Bus Selector2/1 -> Power/2(BodyCg)  "<BdyFrm>"
  Bus Selector1/1 -> Power/1(InertCg)  "<InertFrm>"
  [InfoBus] -> Bus Selector2/1, Bus Selector1/1
  Lateral 3DOF/3(PwrInfo) -> Bus Creator17/3  "PwrInfo"
  Xo/1 -> state2bus/3(Xo)
  Vector Concatenate1/1 -> Lateral 3DOF/7(WhlAngR)
  Vector Concatenate/1 -> Lateral 3DOF/6(WhlAngF)
  WhlAngF/1 -> Vector Concatenate/1, Vector Concatenate/2
  WhlAngR/1 -> Vector Concatenate1/1, Vector Concatenate1/2
  state2bus/2(COM_B) -> Lateral 3DOF/2(BdyFrmCg)  "BdyFrmCg"
  state2bus/1(COM_I) -> Lateral 3DOF/1(InertCg), Bus Selector/1  "InertCg"
  Lateral 3DOF/1(InertFrm) -> Bus Creator17/1  "InertFrm"
  Bus Creator17/1 -> Info/1, [InfoBus]  "Info"
  y/1 -> state2bus/2(y)
  Selector/1 -> Demux/1
  Demux/1 -> Signal Specification15/1
  Demux/2 -> Signal Specification1/1
  Demux/3 -> Signal Specification2/1
  x/1 -> Selector/1, state2bus/1(x)
  Signal Specification15/1 -> xdot/1
  Signal Specification1/1 -> ydot/1
  Signal Specification2/1 -> r/1
  Lateral 3DOF/2(BdyFrm) -> Bus Creator17/2  "BdyFrm"
  Fg/1 -> Forces 3DOF/3(Fg)
  FTire/1 -> Forces 3DOF/6(FTire)
  Forces 3DOF/1(Forces) -> Lateral 3DOF/3(Forces), Power/3(Forces)  "Forces"
  FOut/1 -> Forces 3DOF/4(Fs)
  Forces 3DOF/2(FzF) -> FzF/1
  Forces 3DOF/3(FzR) -> FzR/1
  FExt/1 -> Forces 3DOF/5(Fext)
  Moments/1(Moments) -> Lateral 3DOF/5(Moments), Power/4(Moments)  "Moments"
  MExt/1 -> Moments/3(MExt)  "Ext"
  Power/1(Pwr) -> Lateral 3DOF/4(Power)
  Fbody/1 -> Forces 3DOF/1(FBody)
  MDrag/1 -> Moments/2(Mdrag)  "Drag"
  MTotal/1 -> Moments/1(MBody)

== system PassVeh7DOF/Vehicle Body 3DOF External Longitudinal Wheels/Bicycle/Vehicle Body 3DOF Single Track/Signal Routing/Signal Routing Dual ==
  y : Inport
  Fbody : Inport  Port=2
  MTotal : Inport  Port=3
  FOut : Inport  Port=4
  FTire : Inport  Port=5
  Fg : Inport  Port=6
  FDrag : Inport  Port=7
  MDrag : Inport  Port=8
  FExt : Inport  Port=9
  MExt : Inport  Port=10
  x : Inport  Port=11
  WhlAngF : Inport  Port=12
  WhlAngR : Inport  Port=13
  Fh : Inport  Port=14
  Mh : Inport  Port=15
  Xo : Inport  Port=16
  Bus Creator17 : BusCreator  Inputs=3
  Bus Selector : BusSelector  OutputSignals=Ang.psi
  Bus Selector1 : BusSelector  OutputSignals=InertFrm
  Bus Selector2 : BusSelector  OutputSignals=BdyFrm
  Demux : Demux  Outputs=3
  Forces 3DOF : Subsystem  VariantControl=2
  Ground : Ground
  Lateral 3DOF : Subsystem  VariantControl=2
  Moments : Subsystem
  Power : Subsystem  VariantControl=4
  Selector : Selector  IndexOptions=Index vector (dialog)  Indices=[1,2,4]  OutputSizes=1
  Signal Specification1 : SignalSpecification  Unit=m/s
  Signal Specification15 : SignalSpecification  Unit=m/s
  Signal Specification2 : SignalSpecification  Unit=rad/s
  state2bus : Subsystem
  Info : Outport  VectorParamsAs1DForOutWhenUnconnected=off
  xdot : Outport  Port=2  VectorParamsAs1DForOutWhenUnconnected=off
  ydot : Outport  Port=3  VectorParamsAs1DForOutWhenUnconnected=off
  psi : Outport  Port=4  VectorParamsAs1DForOutWhenUnconnected=off
  r : Outport  Port=5  VectorParamsAs1DForOutWhenUnconnected=off
  FzF : Outport  Port=6  VectorParamsAs1DForOutWhenUnconnected=off
  FzR : Outport  Port=7  VectorParamsAs1DForOutWhenUnconnected=off
  wires:
  Fh/1 -> Forces 3DOF/7(Fh)
  FTire/1 -> Forces 3DOF/6(FTire)
  Mh/1 -> Moments/4(Mh)  "Mh"
  Bus Selector/1 -> psi/1  "<psi>"
  Demux/3 -> Signal Specification2/1
  Ground/1 -> Power/5(Fsusp)
  Lateral 3DOF/3(PwrInfo) -> Bus Creator17/3  "PwrInfo"
  Bus Selector1/1 -> Power/1(InertCg)  "<InertFrm>"
  [InfoBus] -> Bus Selector2/1, Bus Selector1/1
  Bus Selector2/1 -> Power/2(BodyCg)  "<BdyFrm>"
  Xo/1 -> state2bus/3(Xo)
  WhlAngR/1 -> Lateral 3DOF/7(WhlAngR)
  WhlAngF/1 -> Lateral 3DOF/6(WhlAngF)
  MTotal/1 -> Moments/1(MBody)
  MDrag/1 -> Moments/2(Mdrag)  "Drag"
  Fbody/1 -> Forces 3DOF/1(FBody)
  Power/1(Pwr) -> Lateral 3DOF/4(Power)
  MExt/1 -> Moments/3(MExt)  "Ext"
  Moments/1(Moments) -> Lateral 3DOF/5(Moments), Power/4(Moments)  "Moments"
  FExt/1 -> Forces 3DOF/5(Fext)
  Forces 3DOF/3(FzR) -> FzR/1
  Forces 3DOF/2(FzF) -> FzF/1
  FDrag/1 -> Forces 3DOF/2(Fdrag)
  FOut/1 -> Forces 3DOF/4(Fs)
  Forces 3DOF/1(Forces) -> Lateral 3DOF/3(Forces), Power/3(Forces)  "Forces"
  Fg/1 -> Forces 3DOF/3(Fg)
  Lateral 3DOF/2(BdyFrm) -> Bus Creator17/2  "BdyFrm"
  Signal Specification2/1 -> r/1
  Signal Specification1/1 -> ydot/1
  Signal Specification15/1 -> xdot/1
  x/1 -> Selector/1, state2bus/1(x)
  state2bus/2(COM_B) -> Lateral 3DOF/2(BdyFrmCg)  "BdyFrmCg"
  state2bus/1(COM_I) -> Bus Selector/1, Lateral 3DOF/1(InertCg)  "InertCg"
  Demux/2 -> Signal Specification1/1
  Demux/1 -> Signal Specification15/1
  Selector/1 -> Demux/1
  y/1 -> state2bus/2(y)
  Bus Creator17/1 -> Info/1, [InfoBus]  "Info"
  Lateral 3DOF/1(InertFrm) -> Bus Creator17/1  "InertFrm"

== system PassVeh7DOF/Vehicle Body 3DOF External Longitudinal Wheels/Bicycle/Vehicle Body 3DOF Single Track/friction/mu ext ==
  mu_in : Inport  Unit=1
  Signal Specification1 : SignalSpecification  Unit=1
  Unit Conversion2 : UnitConversion
  mu_out : Outport  Unit=1  VectorParamsAs1DForOutWhenUnconnected=off
  wires:
  Signal Specification1/1 -> mu_out/1
  mu_in/1 -> Unit Conversion2/1
  Unit Conversion2/1 -> Signal Specification1/1

== system PassVeh7DOF/Vehicle Body 3DOF External Longitudinal Wheels/Bicycle/Vehicle Body 3DOF Single Track/friction/mu ext dual ==
  mu_in : Inport  PortDimensions=[2,2]
  Signal Specification1 : SignalSpecification  Unit=1
  Unit Conversion2 : UnitConversion
  mu_out : Outport  PortDimensions=[2,2]  VectorParamsAs1DForOutWhenUnconnected=off
  wires:
  Signal Specification1/1 -> mu_out/1
  mu_in/1 -> Unit Conversion2/1
  Unit Conversion2/1 -> Signal Specification1/1

== system PassVeh7DOF/Vehicle Body 3DOF External Longitudinal Wheels/Bicycle/Vehicle Body 3DOF Single Track/friction/mu int ==
  Constant : Constant  Value=mu
  Vector Concatenate1 : Concatenate
  mu_out : Outport  VectorParamsAs1DForOutWhenUnconnected=off
  wires:
  Constant/1 -> Vector Concatenate1/1, Vector Concatenate1/2
  Vector Concatenate1/1 -> mu_out/1

== system PassVeh7DOF/Vehicle Body 3DOF External Longitudinal Wheels/Bicycle/Vehicle Body 3DOF Single Track/friction/mu int dual ==
  Constant : Constant  Value=mu
  Vector Concatenate2 : Concatenate  Mode=Multidimensional array  ConcatenateDimension=2
  Vector Concatenate3 : Concatenate  Mode=Multidimensional array  ConcatenateDimension=2
  Vector Concatenate4 : Concatenate  Mode=Multidimensional array
  mu_out : Outport  VectorParamsAs1DForOutWhenUnconnected=off
  wires:
  Vector Concatenate2/1 -> Vector Concatenate4/1
  Vector Concatenate3/1 -> Vector Concatenate4/2
  Vector Concatenate4/1 -> mu_out/1
  Constant/1 -> Vector Concatenate3/2, Vector Concatenate3/1, Vector Concatenate2/2, Vector Concatenate2/1

== system PassVeh7DOF/Vehicle Body 3DOF External Longitudinal Wheels/Bicycle/Vehicle Body 3DOF Single Track/front forces/ext ==
  F_in : Inport  PortDimensions=2
  Signal Specification1 : SignalSpecification  Unit=N
  Unit Conversion3 : UnitConversion
  F_out : Outport  Unit=N  VectorParamsAs1DForOutWhenUnconnected=off
  wires:
  Signal Specification1/1 -> F_out/1
  F_in/1 -> Unit Conversion3/1
  Unit Conversion3/1 -> Signal Specification1/1

== system PassVeh7DOF/Vehicle Body 3DOF External Longitudinal Wheels/Bicycle/Vehicle Body 3DOF Single Track/front forces/ext dual ==
  F_in : Inport  PortDimensions=[2,2]
  Signal Specification1 : SignalSpecification  Unit=N
  Unit Conversion3 : UnitConversion
  F_out : Outport  Unit=N  PortDimensions=[2,2]  VectorParamsAs1DForOutWhenUnconnected=off
  wires:
  Signal Specification1/1 -> F_out/1
  F_in/1 -> Unit Conversion3/1
  Unit Conversion3/1 -> Signal Specification1/1

== system PassVeh7DOF/Vehicle Body 3DOF External Longitudinal Wheels/Bicycle/Vehicle Body 3DOF Single Track/front forces/ext long ==
  F_in : Inport
  Ground1 : Ground
  Signal Specification : SignalSpecification  Unit=N
  Signal Specification1 : SignalSpecification  Unit=N
  Unit Conversion1 : UnitConversion
  Vector Concatenate1 : Concatenate
  F_out : Outport  Unit=N  VectorParamsAs1DForOutWhenUnconnected=off
  wires:
  Signal Specification/1 -> Vector Concatenate1/2
  F_in/1 -> Unit Conversion1/1
  Vector Concatenate1/1 -> F_out/1
  Ground1/1 -> Signal Specification/1
  Unit Conversion1/1 -> Signal Specification1/1
  Signal Specification1/1 -> Vector Concatenate1/1

== system PassVeh7DOF/Vehicle Body 3DOF External Longitudinal Wheels/Bicycle/Vehicle Body 3DOF Single Track/front forces/ext long dual ==
  F_in : Inport
  Demux : Demux  Outputs=2
  Ground : Ground
  Signal Specification5 : SignalSpecification  Unit=N
  Unit Conversion2 : UnitConversion  OutputType=Inherit: Inherit via back propagation
  Vector Concatenate1 : Concatenate  Mode=Multidimensional array  ConcatenateDimension=2
  Vector Concatenate2 : Concatenate  Mode=Multidimensional array  ConcatenateDimension=2
  Vector Concatenate3 : Concatenate  Mode=Multidimensional array
  F_out : Outport  Unit=N  VectorParamsAs1DForOutWhenUnconnected=off
  wires:
  Ground/1 -> Vector Concatenate2/2, Vector Concatenate1/2
  Vector Concatenate3/1 -> F_out/1
  Vector Concatenate1/1 -> Vector Concatenate3/1
  Vector Concatenate2/1 -> Vector Concatenate3/2
  Demux/1 -> Vector Concatenate1/1
  Demux/2 -> Vector Concatenate2/1
  Unit Conversion2/1 -> Signal Specification5/1
  Signal Specification5/1 -> Demux/1
  F_in/1 -> Unit Conversion2/1

== system PassVeh7DOF/Vehicle Body 3DOF External Longitudinal Wheels/Bicycle/Vehicle Body 3DOF Single Track/front forces/int ==
  Ground : Ground
  Vector Concatenate1 : Concatenate
  F_out : Outport  VectorParamsAs1DForOutWhenUnconnected=off
  wires:
  Ground/1 -> Vector Concatenate1/2, Vector Concatenate1/1
  Vector Concatenate1/1 -> F_out/1

== system PassVeh7DOF/Vehicle Body 3DOF External Longitudinal Wheels/Bicycle/Vehicle Body 3DOF Single Track/front forces/int dual ==
  Ground : Ground
  Vector Concatenate2 : Concatenate  Mode=Multidimensional array  ConcatenateDimension=2
  Vector Concatenate3 : Concatenate  Mode=Multidimensional array  ConcatenateDimension=2
  Vector Concatenate4 : Concatenate  Mode=Multidimensional array
  F_out : Outport  VectorParamsAs1DForOutWhenUnconnected=off
  wires:
  Vector Concatenate2/1 -> Vector Concatenate4/1
  Vector Concatenate3/1 -> Vector Concatenate4/2
  Vector Concatenate4/1 -> F_out/1
  Ground/1 -> Vector Concatenate3/2, Vector Concatenate3/1, Vector Concatenate2/2, Vector Concatenate2/1

== system PassVeh7DOF/Vehicle Body 3DOF External Longitudinal Wheels/Bicycle/Vehicle Body 3DOF Single Track/front steer/delta ext ==
  delta_in : Inport  Unit=rad
  Signal Specification1 : SignalSpecification  Unit=rad
  Unit Conversion1 : UnitConversion
  delta_out : Outport  VectorParamsAs1DForOutWhenUnconnected=off
  wires:
  Signal Specification1/1 -> delta_out/1
  Unit Conversion1/1 -> Signal Specification1/1
  delta_in/1 -> Unit Conversion1/1

== system PassVeh7DOF/Vehicle Body 3DOF External Longitudinal Wheels/Bicycle/Vehicle Body 3DOF Single Track/front steer/delta ext dual ==
  delta_in : Inport  PortDimensions=2
  Signal Specification1 : SignalSpecification  Unit=rad
  Unit Conversion2 : UnitConversion
  delta_out : Outport  Unit=rad  PortDimensions=2  VectorParamsAs1DForOutWhenUnconnected=off
  wires:
  Signal Specification1/1 -> delta_out/1
  Unit Conversion2/1 -> Signal Specification1/1
  delta_in/1 -> Unit Conversion2/1

== system PassVeh7DOF/Vehicle Body 3DOF External Longitudinal Wheels/Bicycle/Vehicle Body 3DOF Single Track/front steer/delta int ==
  Ground : Ground
  delta_out : Outport  VectorParamsAs1DForOutWhenUnconnected=off
  wires:
  Ground/1 -> delta_out/1

== system PassVeh7DOF/Vehicle Body 3DOF External Longitudinal Wheels/Bicycle/Vehicle Body 3DOF Single Track/front steer/delta int dual ==
  Constant : Constant  Value=0
  Vector Concatenate4 : Concatenate
  delta_out : Outport  VectorParamsAs1DForOutWhenUnconnected=off
  wires:
  Constant/1 -> Vector Concatenate4/1, Vector Concatenate4/2
  Vector Concatenate4/1 -> delta_out/1

== system PassVeh7DOF/Vehicle Body 3DOF External Longitudinal Wheels/Bicycle/Vehicle Body 3DOF Single Track/hitch geometry parameters/hitch active bicycle ==
  Constant : Constant  Value=dh
  Constant1 : Constant  Value=hh
  Ground : Ground
  dh_out : Outport  VectorParamsAs1DForOutWhenUnconnected=off
  hh_out : Outport  Port=2  VectorParamsAs1DForOutWhenUnconnected=off
  hl_out : Outport  Port=3  VectorParamsAs1DForOutWhenUnconnected=off
  wires:
  Ground/1 -> hl_out/1
  Constant1/1 -> hh_out/1
  Constant/1 -> dh_out/1

== system PassVeh7DOF/Vehicle Body 3DOF External Longitudinal Wheels/Bicycle/Vehicle Body 3DOF Single Track/hitch geometry parameters/hitch active dual track ==
  Constant : Constant  Value=dh
  Constant1 : Constant  Value=hh
  Constant2 : Constant  Value=hl
  dh_out : Outport  VectorParamsAs1DForOutWhenUnconnected=off
  hh_out : Outport  Port=2  VectorParamsAs1DForOutWhenUnconnected=off
  hl_out : Outport  Port=3  VectorParamsAs1DForOutWhenUnconnected=off
  wires:
  Constant2/1 -> hl_out/1
  Constant1/1 -> hh_out/1
  Constant/1 -> dh_out/1

== system PassVeh7DOF/Vehicle Body 3DOF External Longitudinal Wheels/Bicycle/Vehicle Body 3DOF Single Track/hitch geometry parameters/hitch inactive ==
  Ground : Ground
  dh_out : Outport  Unit=m  PortDimensions=1  VectorParamsAs1DForOutWhenUnconnected=off
  hh_out : Outport  Port=2  Unit=m  PortDimensions=1  VectorParamsAs1DForOutWhenUnconnected=off
  hl_out : Outport  Port=3  Unit=m  PortDimensions=1  VectorParamsAs1DForOutWhenUnconnected=off
  wires:
  Ground/1 -> dh_out/1, hh_out/1, hl_out/1

== system PassVeh7DOF/Vehicle Body 3DOF External Longitudinal Wheels/Bicycle/Vehicle Body 3DOF Single Track/rear forces/ext ==
  F_in : Inport  PortDimensions=2
  Signal Specification1 : SignalSpecification  Unit=N
  Unit Conversion3 : UnitConversion
  F_out : Outport  Unit=N  VectorParamsAs1DForOutWhenUnconnected=off
  wires:
  Signal Specification1/1 -> F_out/1
  F_in/1 -> Unit Conversion3/1
  Unit Conversion3/1 -> Signal Specification1/1

== system PassVeh7DOF/Vehicle Body 3DOF External Longitudinal Wheels/Bicycle/Vehicle Body 3DOF Single Track/rear forces/ext dual ==
  F_in : Inport  PortDimensions=[2,2]
  Signal Specification1 : SignalSpecification  Unit=N
  Unit Conversion3 : UnitConversion
  F_out : Outport  Unit=N  PortDimensions=[2,2]  VectorParamsAs1DForOutWhenUnconnected=off
  wires:
  Signal Specification1/1 -> F_out/1
  F_in/1 -> Unit Conversion3/1
  Unit Conversion3/1 -> Signal Specification1/1

== system PassVeh7DOF/Vehicle Body 3DOF External Longitudinal Wheels/Bicycle/Vehicle Body 3DOF Single Track/rear forces/ext long ==
  F_in : Inport
  Ground1 : Ground
  Signal Specification : SignalSpecification  Unit=N
  Signal Specification1 : SignalSpecification  Unit=N
  Unit Conversion1 : UnitConversion
  Vector Concatenate1 : Concatenate
  F_out : Outport  Unit=N  VectorParamsAs1DForOutWhenUnconnected=off
  wires:
  Signal Specification/1 -> Vector Concatenate1/2
  F_in/1 -> Unit Conversion1/1
  Vector Concatenate1/1 -> F_out/1
  Ground1/1 -> Signal Specification/1
  Unit Conversion1/1 -> Signal Specification1/1
  Signal Specification1/1 -> Vector Concatenate1/1

== system PassVeh7DOF/Vehicle Body 3DOF External Longitudinal Wheels/Bicycle/Vehicle Body 3DOF Single Track/rear forces/ext long dual ==
  F_in : Inport
  Demux : Demux  Outputs=2
  Ground : Ground
  Signal Specification5 : SignalSpecification  Unit=N
  Unit Conversion2 : UnitConversion  OutputType=Inherit: Inherit via back propagation
  Vector Concatenate1 : Concatenate  Mode=Multidimensional array  ConcatenateDimension=2
  Vector Concatenate2 : Concatenate  Mode=Multidimensional array  ConcatenateDimension=2
  Vector Concatenate3 : Concatenate  Mode=Multidimensional array
  F_out : Outport  Unit=N  VectorParamsAs1DForOutWhenUnconnected=off
  wires:
  Ground/1 -> Vector Concatenate2/2, Vector Concatenate1/2
  Vector Concatenate3/1 -> F_out/1
  Vector Concatenate1/1 -> Vector Concatenate3/1
  Vector Concatenate2/1 -> Vector Concatenate3/2
  Demux/1 -> Vector Concatenate1/1
  Demux/2 -> Vector Concatenate2/1
  Unit Conversion2/1 -> Signal Specification5/1
  Signal Specification5/1 -> Demux/1
  F_in/1 -> Unit Conversion2/1

== system PassVeh7DOF/Vehicle Body 3DOF External Longitudinal Wheels/Bicycle/Vehicle Body 3DOF Single Track/rear forces/int ==
  Ground : Ground
  Vector Concatenate1 : Concatenate
  F_out : Outport  VectorParamsAs1DForOutWhenUnconnected=off
  wires:
  Ground/1 -> Vector Concatenate1/2, Vector Concatenate1/1
  Vector Concatenate1/1 -> F_out/1

== system PassVeh7DOF/Vehicle Body 3DOF External Longitudinal Wheels/Bicycle/Vehicle Body 3DOF Single Track/rear forces/int dual ==
  Ground : Ground
  Vector Concatenate2 : Concatenate  Mode=Multidimensional array  ConcatenateDimension=2
  Vector Concatenate3 : Concatenate  Mode=Multidimensional array  ConcatenateDimension=2
  Vector Concatenate4 : Concatenate  Mode=Multidimensional array
  F_out : Outport  VectorParamsAs1DForOutWhenUnconnected=off
  wires:
  Vector Concatenate2/1 -> Vector Concatenate4/1
  Vector Concatenate3/1 -> Vector Concatenate4/2
  Vector Concatenate4/1 -> F_out/1
  Ground/1 -> Vector Concatenate3/2, Vector Concatenate3/1, Vector Concatenate2/2, Vector Concatenate2/1

== system PassVeh7DOF/Vehicle Body 3DOF External Longitudinal Wheels/Bicycle/Vehicle Body 3DOF Single Track/rear steer/delta ext ==
  delta_in : Inport  Unit=rad
  Signal Specification1 : SignalSpecification  Unit=rad
  Unit Conversion1 : UnitConversion
  delta_out : Outport  VectorParamsAs1DForOutWhenUnconnected=off
  wires:
  Signal Specification1/1 -> delta_out/1
  Unit Conversion1/1 -> Signal Specification1/1
  delta_in/1 -> Unit Conversion1/1
